simulink model "micro2018b"  (R2018b)
settings: Solver=ode1  StartTime=0.0  StopTime=t_sim  FixedStep=Ts  RelTol=1e-3
values from neighbouring files (symbols this model uses):
  Vo = 200    [param.m]
undefined symbols (not defined in the file or in its folder): C, f_i, fo, L, L1, L2, phi, R, Tm, Ts, Vac_pk
libraries: powerlib x16, powerlib_meascontrol x2, simulink x1, hdlsllib x1
(part 1 of 2)
settings Model: Creator=gomez  LastModifiedBy=gomez
settings DataIOCC: ReturnWorkspaceOutputs=on
settings DebuggingCC: UnconnectedInputMsg=none  UnconnectedOutputMsg=none  UnconnectedLineMsg=none  SFMachineParentedDataDiag=error

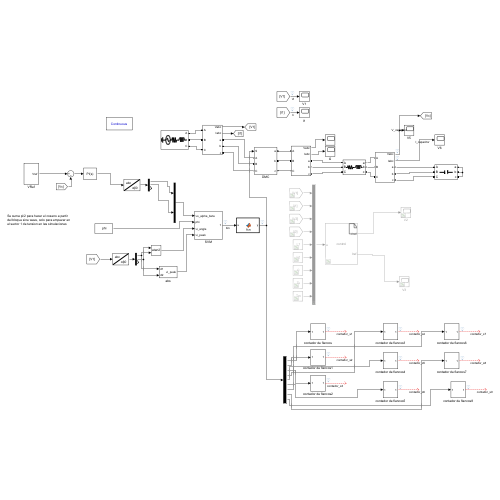
[thumbnail: Simulink's stored preview of the top-level diagram]
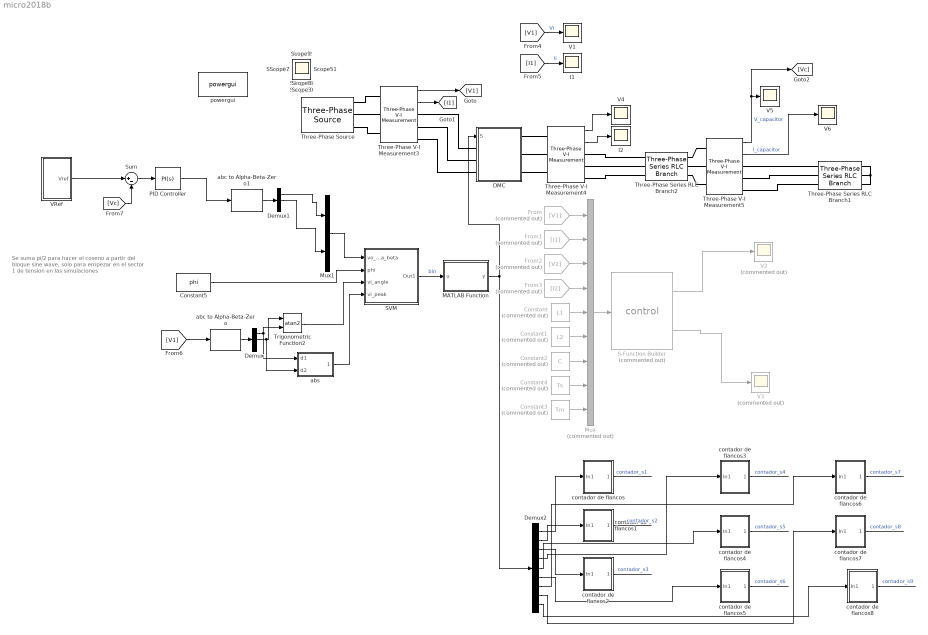
== system micro2018b ==
  note: Se suma pi/2 para hacer el coseno a partir del bloque sine wave, solo para empezar en el sector 1 de tension en las simulaciones
  Constant : Constant  Commented=on  Value=L1
  Constant1 : Constant  Commented=on  Value=L2
  Constant2 : Constant  Commented=on  Value=C
  Constant3 : Constant  Commented=on  Value=Tm
  Constant4 : Constant  Commented=on  Value=Ts
  Constant5 : Constant  Value=phi
  DMC : Subsystem
  Demux : Demux  Outputs=3
  Demux1 : Demux  Outputs=3
  Demux2 : Demux  Outputs=9
  From : From  Commented=on  GotoTag=V1
  From1 : From  Commented=on  GotoTag=I1
  From2 : From  Commented=on  GotoTag=V2
  From3 : From  Commented=on  GotoTag=I2
  I1 : Scope
  I2 : Scope
  MATLAB Function : MATLAB Function  TreatAsAtomicUnit=on
  Mux : Mux  Commented=on  Inputs=9
  Mux1 : Mux  Inputs=2
  PID Controller : simulink/Continuous/PID Controller  Controller=PI  Form=Parallel  TimeDomain=Continuous-time  SampleTime=-1  IntegratorMethod=Forward Euler  ControllerParametersSource=internal  P=1  I=1  D=0  N=100  UseFilter=on  TunerSelectOption=Transfer Function Based (PID Tuner App)  InitialConditionSource=internal  InitialConditionForIntegrator=0  InitialConditionForFilter=0  DifferentiatorICPrevScaledInput=0  ExternalReset=none  TrackingMode=off  Kt=1  LimitOutput=off  UpperSaturationLimit=inf  LowerSaturationLimit=-inf  LinearizeAsGain=on  AntiWindupMode=none  Kb=1  POutMin=[]  POutMax=[]  IOutMin=[]  IOutMax=[]  DOutMin=[]  DOutMax=[]  NOutMin=[]  NOutMax=[]  SumOutMin=[]  SumOutMax=[]  SaturationOutMin=[]  SaturationOutMax=[]  PParamMin=[]  PParamMax=[]  IParamMin=[]  IParamMax=[]  DParamMin=[]  DParamMax=[]  NParamMin=[]  NParamMax=[]  KbParamMin=[]  KbParamMax=[]  KtParamMin=[]  KtParamMax=[]  KbOutMin=[]  KbOutMax=[]  KtOutMin=[]  KtOutMax=[]  IntegratorOutMin=[]  IntegratorOutMax=[]  FilterOutMin=[]  FilterOutMax=[]  SumI1OutMin=[]  SumI1OutMax=[]  SumI2OutMin=[]  SumI2OutMax=[]  SumI3OutMin=[]  SumI3OutMax=[]  SumI4OutMin=[]  SumI4OutMax=[]  SumDOutMin=[]  SumDOutMax=[]  DifferentiatorOutMin=[]  DifferentiatorOutMax=[]  FilterDiffOutCoefMin=[]  FilterDiffOutCoefMax=[]  ReciprocalOutMin=[]  ReciprocalOutMax=[]  SumDenOutMin=[]  SumDenOutMax=[]  SumNumOutMin=[]  SumNumOutMax=[]  DivideOutMin=[]  DivideOutMax=[]  IntegratorContinuousStateAttributes=''  IntegratorStateMustResolveToSignalObject=off  IntegratorRTWStateStorageClass=Auto  FilterContinuousStateAttributes=''  FilterStateMustResolveToSignalObject=off  FilterRTWStateStorageClass=Auto  ParallelPVariant=InternalParameters  IdealPVariant=Disabled  IVariant=InternalParameters  DVariant=Disabled  IntegratorVariant=Continuous  SatVariant=Disabled  AWVariant=Passthrough  PCopyVariant=Disabled  TRVariant=Disabled  FdbkBlocksVariant=Forward  IdealPFdbkVariant=Disabled  SatFdbkVariant=Disabled  DerivativeFilterVariant=Disabled  NVariant=Disabled  NCopyVariant=Disabled_SignalSpec  FilterICVariant=Disabled  IntegratorICVariant=InternalICs  ExternalResetVariant=Disabled  TRSumVariant=Passthrough  SumFdbkVariant=Disabled  SumVariant=Sum_PI
  S-Function Builder : S-Function  Commented=on  FunctionName=control  SFunctionModules=control_wrapper  SFunctionDeploymentMode=off  EnableBusSupport=off  mask(S-Function Builder){}
      mask help: Simulink:masks:SFunctionBuilder_MD
      mask init:
      | val = [[.9  0.75 0.75 1 1 .9 .9 1]',[1 1 0.75 0.75 .9 .9 1 .9]'];try , sys = get_param(gcb,'SfunBuilderFcnName');if isempty(sys), sys = get_param(gcb,'FunctionName'); end,catch, sys = get_param(gcb,'FunctionName'); end
      settings: CopyFcn=set_param(gcbh,'LinkStatus','none')  OpenFcn=sfunctionwizard(gcbh)
      mask Display:
      | plot(val(:,1),val(:,2))
      | disp(sys)
      | port_label('input',1,'u')
      | port_label('output',1,'Vref')
      | port_label('output',2,'Iref')
  SVM : Subsystem
  Sum : Sum  Inputs=|+-
  Three-Phase Series RLC Branch1 : powerlib/Elements/Three-Phase Series RLC Branch  LConnTagsString=A|B|C  RConnTagsString=A|B|C  BranchType=C  Resistance=R  Inductance=L  Capacitance=C  Measurements=None
  Three-Phase Series RLC Branch2 : powerlib/Elements/Three-Phase Series RLC Branch  LConnTagsString=A|B|C  RConnTagsString=A|B|C  BranchType=RL  Resistance=R  Inductance=L  Capacitance=C  Measurements=None
  Three-Phase V-I Measurement3 : powerlib/Measurements/Three-Phase V-I Measurement  VoltageMeasurement=phase-to-ground  SetLabelV=off  LabelV=Vabc  Vpu=off  VpuLL=off  CurrentMeasurement=yes  SetLabelI=off  LabelI=Iabc  Ipu=off  Pbase=100e6  Vbase=500e3  OutputType=Complex  PhasorSimulation=off  PSBequivalent=0
  Three-Phase V-I Measurement4 : powerlib/Measurements/Three-Phase V-I Measurement  VoltageMeasurement=phase-to-ground  SetLabelV=off  LabelV=Vabc  Vpu=off  VpuLL=off  CurrentMeasurement=yes  SetLabelI=off  LabelI=Iabc  Ipu=off  Pbase=100e6  Vbase=500e3  OutputType=Complex  PhasorSimulation=off  PSBequivalent=0
  Three-Phase V-I Measurement5 : powerlib/Measurements/Three-Phase V-I Measurement  VoltageMeasurement=phase-to-ground  SetLabelV=off  LabelV=Vabc  Vpu=off  VpuLL=off  CurrentMeasurement=yes  SetLabelI=off  LabelI=Iabc  Ipu=off  Pbase=100e6  Vbase=500e3  OutputType=Complex  PhasorSimulation=off  PSBequivalent=0
  Three-Phase Source : powerlib/Electrical Sources/Three-Phase Source  InternalConnection=Yg  VoltagePhases=off  Voltage=Vac_pk  PhaseAngle=0  Voltage_phases=[25e3 25e3 25e3]/sqrt(3)  PhaseAngles_phases=[0 -120 +120]  Frequency=f_i  NonIdealSource=on  SpecifyImpedance=off  Resistance=0.1  Inductance=1e-3  ShortCircuitLevel=100e6  BaseVoltage=25e3  XRratio=7  BusType=swing  Pref=10e3  Qref=0  Prefabc=[10e3, 10e3, 10e3]  Qrefabc=[0, 0, 0]  Qmin=-inf  Qmax=inf
  Trigonometric Function2 : Trigonometry  Operator=atan2
  V{1,4..6} (4 alike) : Scope
  V2 : Scope  Commented=on
  V3 : Scope  Commented=on
  VRef : Subsystem
  abc to Alpha-Beta-Zero : powerlib_meascontrol/Transformations/abc to Alpha-Beta-Zero
  abc to Alpha-Beta-Zero1 : powerlib_meascontrol/Transformations/abc to Alpha-Beta-Zero
  abs : Subsystem
  contador de flancos : Subsystem
  contador de flancos1 : Subsystem
  contador de flancos2 : Subsystem
  contador de flancos3 : Subsystem
  contador de flancos4 : Subsystem
  contador de flancos5 : Subsystem
  contador de flancos6 : Subsystem
  contador de flancos7 : Subsystem
  contador de flancos8 : Subsystem
  powergui : powerlib/powergui  Priority=1  SimulationMode=Continuous  SampleTime=50e-6  frequency=60  Iterations=50  frequencyindice=50  Pbase=100e6  ErrMax=1e-4  UnitsV=kV  UnitsW=MW  buscounter=0  FunctionMessages=off  echomessages=off  EnableUseOfTLC=off  CurrentSourceSwitches=off  DisableSnubberDevices=off  DisableRonSwitches=off  DisableVfSwitches=off  DisplayEquations=off  AutomaticDiscreteSolvers=off  SolverType=Tustin/Backward Euler (TBE)  Interpol=off  ExternalGateDelay=off  methode=off  Ts=100  x0status=blocks  SPID=on  SwTol=0  HookPort=off  NonlinearTolerance=1e-4  nMaxIteration=100  ContinueOnMaxIteration=off  RestoreLinks=warning  ResistiveCurrentMeasurement=off  Frange=[0:2:500]  Ylog=off  Xlog=on  ShowGrid=off  save=off  variable=ZData  structure=0  ZoomFFT=off  StartTime=0.0  cycles=1  DisplayStyle=1  fundamental=60  FreqAxis=off  MaxFrequency=1000  frequencyindicesteady=1  RmsSteady=1  display=off
  Scope{,1..3,5,7..13} (12 alike) : Scope
  wires:
  Mux/1 -> S-Function Builder/1
  From/1 -> Mux/1
  From1/1 -> Mux/2
  From2/1 -> Mux/3
  From3/1 -> Mux/4
  Constant/1 -> Mux/5
  Constant1/1 -> Mux/6
  Constant2/1 -> Mux/7
  Constant4/1 -> Mux/8
  Constant3/1 -> Mux/9
  [V1] -> V1/1  "Vi"
  [I1] -> I1/1  "Ii"
  S-Function Builder/1 -> V2/1
  S-Function Builder/2 -> V3/1
  Constant5/1 -> SVM/2(phi)
  Demux1/1 -> Mux1/1
  Demux1/2 -> Mux1/2
  Mux1/1 -> SVM/1(vo_alpha_beta)
  SVM/1(Out1) -> MATLAB Function/1(u)  "bin"
  [V1] -> abc to Alpha-Beta-Zero/1
  abc to Alpha-Beta-Zero/1 -> Demux/1
  Demux/2 -> abs/2(d2), Trigonometric Function2/1
  Demux/1 -> Trigonometric Function2/2, abs/1(d1)
  Trigonometric Function2/1 -> SVM/3(vi_angle)
  abs/1(vi_peak) -> SVM/4(vi_peak)
  Three-Phase V-I Measurement4/1 -> V4/1
  Three-Phase V-I Measurement4/2 -> I2/1
  MATLAB Function/1(y) -> Demux2/1, DMC/1(S)
  Three-Phase V-I Measurement3/1 -> [V1]
  Three-Phase V-I Measurement3/2 -> [I1]
  Three-Phase V-I Measurement5/1 -> [Vc], V5/1  "V_capacitor"
  Three-Phase V-I Measurement5/2 -> V6/1  "I_capacitor"
  abc to Alpha-Beta-Zero1/1 -> Demux1/1
  Demux2/1 -> contador de flancos/1(In1)
  contador de flancos/1(Out1) -> ?  "contador_s1"
  contador de flancos1/1(Out1) -> ?  "contador_s2"
  Demux2/2 -> contador de flancos1/1(In1)
  contador de flancos2/1(Out1) -> ?  "contador_s3"
  Demux2/3 -> contador de flancos2/1(In1)
  contador de flancos3/1(Out1) -> ?  "contador_s4"
  Demux2/4 -> contador de flancos3/1(In1)
  contador de flancos4/1(Out1) -> ?  "contador_s5"
  Demux2/5 -> contador de flancos4/1(In1)
  contador de flancos5/1(Out1) -> ?  "contador_s6"
  Demux2/6 -> contador de flancos5/1(In1)
  contador de flancos6/1(Out1) -> ?  "contador_s7"
  Demux2/7 -> contador de flancos6/1(In1)
  contador de flancos7/1(Out1) -> ?  "contador_s8"
  Demux2/8 -> contador de flancos7/1(In1)
  contador de flancos8/1(Out1) -> ?  "contador_s9"
  Demux2/9 -> contador de flancos8/1(In1)
  VRef/1(Vref) -> Sum/1
  [Vc] -> Sum/2
  Sum/1 -> PID Controller/1
  PID Controller/1 -> abc to Alpha-Beta-Zero1/1
  connections:
  Three-Phase V-I Measurement4/RConn1 -- Three-Phase Series RLC Branch2/LConn1
  Three-Phase Source/RConn1 -- Three-Phase V-I Measurement3/LConn1
  Three-Phase Source/RConn3 -- Three-Phase V-I Measurement3/LConn3
  Three-Phase V-I Measurement4/LConn1 -- DMC/RConn1
  Three-Phase V-I Measurement4/LConn2 -- DMC/RConn2
  Three-Phase V-I Measurement4/LConn3 -- DMC/RConn3
  Three-Phase Series RLC Branch2/LConn2 -- Three-Phase V-I Measurement4/RConn2
  Three-Phase Series RLC Branch2/LConn3 -- Three-Phase V-I Measurement4/RConn3
  Three-Phase Source/RConn2 -- Three-Phase V-I Measurement3/LConn2
  Three-Phase V-I Measurement3/RConn2 -- DMC/LConn2
  Three-Phase V-I Measurement3/RConn1 -- DMC/LConn1
  Three-Phase V-I Measurement3/RConn3 -- DMC/LConn3
  Three-Phase V-I Measurement5/RConn1 -- Three-Phase Series RLC Branch1/LConn1
  Three-Phase V-I Measurement5/RConn2 -- Three-Phase Series RLC Branch1/LConn2
  Three-Phase V-I Measurement5/RConn3 -- Three-Phase Series RLC Branch1/LConn3
  Three-Phase Series RLC Branch1/RConn1 -- Three-Phase Series RLC Branch1/RConn2 -- Three-Phase Series RLC Branch1/RConn3
  Three-Phase Series RLC Branch2/RConn2 -- Three-Phase V-I Measurement5/LConn2
  Three-Phase V-I Measurement5/LConn1 -- Three-Phase Series RLC Branch2/RConn1
  Three-Phase V-I Measurement5/LConn3 -- Three-Phase Series RLC Branch2/RConn3

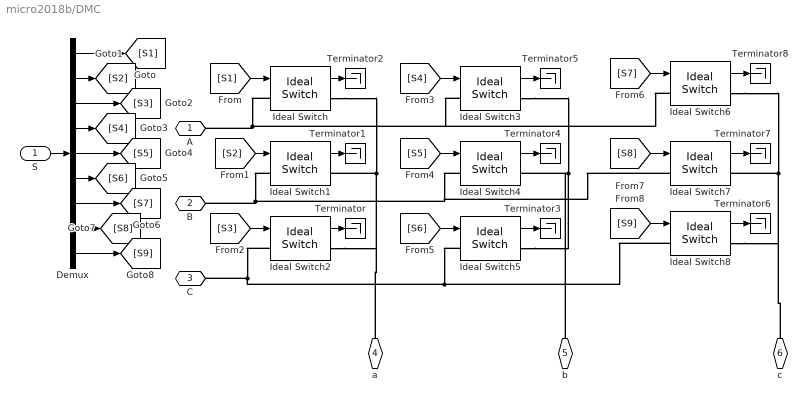
== system micro2018b/DMC ==
  S : Inport
  Demux : Demux  Outputs=9
  Ideal Switch{,1..8} (9 alike) : powerlib/Power Electronics/Ideal Switch  Ron=0.001  Lon=0  IC=0  Rs=1e5  Cs=inf  Measurements=on
  Terminator{,1..8} (9 alike) : Terminator
  A : PMIOPort  Side=Left
  B : PMIOPort  Port=2  Side=Left
  C : PMIOPort  Port=3  Side=Left
  a : PMIOPort  Port=4  Side=Right
  b : PMIOPort  Port=5  Side=Right
  c : PMIOPort  Port=6  Side=Right
  wires:
  [S8] -> Ideal Switch7/1
  Ideal Switch4/1 -> Terminator4/1
  Ideal Switch/1 -> Terminator2/1
  Ideal Switch7/1 -> Terminator7/1
  Ideal Switch8/1 -> Terminator6/1
  Ideal Switch3/1 -> Terminator5/1
  Ideal Switch6/1 -> Terminator8/1
  Ideal Switch2/1 -> Terminator/1
  Ideal Switch1/1 -> Terminator1/1
  [S4] -> Ideal Switch3/1
  [S3] -> Ideal Switch2/1
  Ideal Switch5/1 -> Terminator3/1
  [S2] -> Ideal Switch1/1
  [S9] -> Ideal Switch8/1
  [S6] -> Ideal Switch5/1
  [S5] -> Ideal Switch4/1
  [S1] -> Ideal Switch/1
  Demux/1 -> [S1]
  Demux/2 -> [S2]
  Demux/3 -> [S3]
  Demux/4 -> [S4]
  Demux/5 -> [S5]
  Demux/6 -> [S6]
  Demux/7 -> [S7]
  Demux/8 -> [S8]
  Demux/9 -> [S9]
  [S7] -> Ideal Switch6/1
  S/1 -> Demux/1
  connections:
  Ideal Switch1/LConn1 -- Ideal Switch4/LConn1 -- Ideal Switch7/LConn1 -- B/RConn1
  Ideal Switch/RConn1 -- a/RConn1 -- Ideal Switch2/RConn1 -- Ideal Switch1/RConn1
  Ideal Switch6/RConn1 -- Ideal Switch7/RConn1 -- c/RConn1 -- Ideal Switch8/RConn1
  Ideal Switch8/LConn1 -- Ideal Switch2/LConn1 -- C/RConn1 -- Ideal Switch5/LConn1
  Ideal Switch/LConn1 -- Ideal Switch6/LConn1 -- Ideal Switch3/LConn1 -- A/RConn1
  Ideal Switch3/RConn1 -- b/RConn1 -- Ideal Switch5/RConn1 -- Ideal Switch4/RConn1

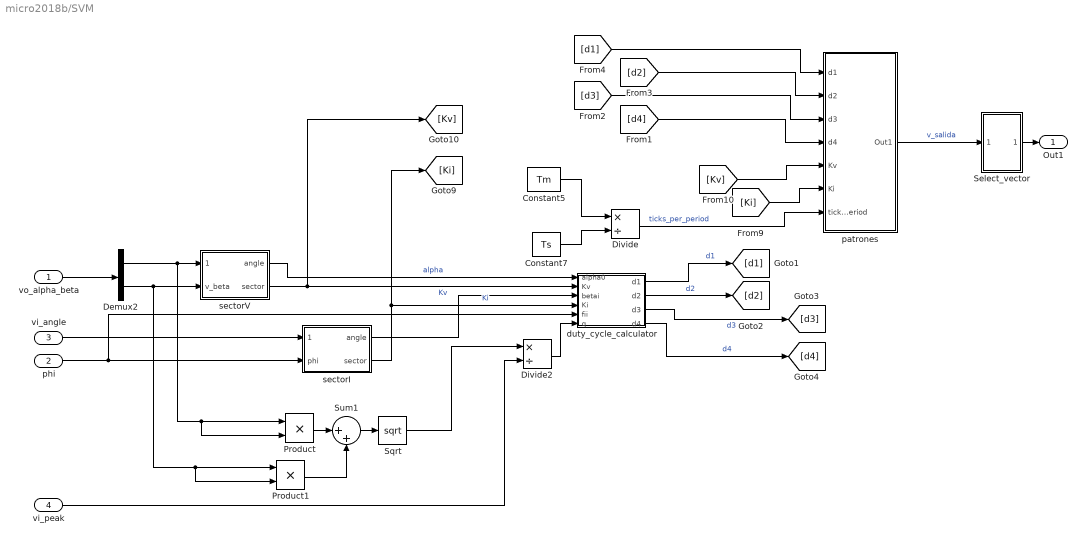
== system micro2018b/SVM ==
  vo_alpha_beta : Inport
  phi : Inport  Port=2
  vi_angle : Inport  Port=3
  vi_peak : Inport  Port=4
  Constant5 : Constant  Value=Tm
  Constant7 : Constant  Value=Ts
  Demux2 : Demux  Outputs=2
  Divide : Product  Inputs=*/
  Divide2 : Product  Inputs=*/
  Product : Product
  Product1 : Product
  Select_vector : Subsystem
  Sqrt : Sqrt  SaturateOnIntegerOverflow=on
  Sum1 : Sum  Inputs=|++
  duty_cycle_calculator : MATLAB Function  TreatAsAtomicUnit=on
  patrones : Subsystem
  sectorI : MATLAB Function  TreatAsAtomicUnit=on
  sectorV : MATLAB Function  TreatAsAtomicUnit=on
  Out1 : Outport
  wires:
  Sqrt/1 -> Divide2/1
  duty_cycle_calculator/4(d4) -> [d4]  "d4"
  sectorV/1(angle) -> duty_cycle_calculator/1(alpha0)  "alpha"
  duty_cycle_calculator/3(d3) -> [d3]  "d3"
  Demux2/2 -> Product1/2, Product1/1, sectorV/2(v_beta)
  vo_alpha_beta/1 -> Demux2/1
  Demux2/1 -> Product/2, Product/1, sectorV/1(v_alpha)
  sectorV/2(sector) -> [Kv], duty_cycle_calculator/2(Kv)  "Kv"
  duty_cycle_calculator/2(d2) -> [d2]  "d2"
  duty_cycle_calculator/1(d1) -> [d1]  "d1"
  Divide2/1 -> duty_cycle_calculator/6(q)
  Product1/1 -> Sum1/2
  phi/1 -> duty_cycle_calculator/5(fii), sectorI/2(phi)
  sectorI/2(sector) -> [Ki], duty_cycle_calculator/4(Ki)  "Ki"
  sectorI/1(angle) -> duty_cycle_calculator/3(betai)
  Sum1/1 -> Sqrt/1
  Product/1 -> Sum1/1
  vi_angle/1 -> sectorI/1(Vi_angle)
  vi_peak/1 -> Divide2/2
  Select_vector/1(Out1) -> Out1/1
  [d1] -> patrones/1(d1)
  [d2] -> patrones/2(d2)
  [d3] -> patrones/3(d3)
  [d4] -> patrones/4(d4)
  [Ki] -> patrones/6(Ki)
  [Kv] -> patrones/5(Kv)
  patrones/1(Out1) -> Select_vector/1(In1)  "v_salida"
  Constant5/1 -> Divide/1
  Constant7/1 -> Divide/2
  Divide/1 -> patrones/7(ticks_per_period)  "ticks_per_period"

== system micro2018b/VRef ==
  Mux : Mux  Inputs=3
  VA : Sin  Amplitude=Vo  Frequency=2*pi*fo  SampleTime=0
  VB : Sin  Amplitude=Vo  Frequency=2*pi*fo  Phase=-2*pi/3  SampleTime=0
  VC : Sin  Amplitude=Vo  Frequency=2*pi*fo  Phase=-4*pi/3  SampleTime=0
  Vref : Outport  VectorParamsAs1DForOutWhenUnconnected=off
  wires:
  VA/1 -> Mux/1
  VB/1 -> Mux/2
  VC/1 -> Mux/3
  Mux/1 -> Vref/1

== system micro2018b/abs ==
  d1 : Inport
  d2 : Inport  Port=2
  Add : Sum
  Product1 : Product
  Product2 : Product
  Sqrt1 : Sqrt  SaturateOnIntegerOverflow=on
  vi_peak : Outport
  wires:
  d1/1 -> Product2/2, Product2/1
  Sqrt1/1 -> vi_peak/1
  d2/1 -> Product1/2, Product1/1
  Product1/1 -> Add/2
  Product2/1 -> Add/1
  Add/1 -> Sqrt1/1

== system micro2018b/contador de flancos ==
  In1 : Inport
  Add : Sum
  Data Type Conversion : DataTypeConversion
  Delay : Delay  DelayLength=1
  Delay1 : Delay  DelayLength=1
  Relational Operator : RelationalOperator  Operator=>  OutDataTypeStr=boolean  RndMeth=Simplest
  Out1 : Outport
  wires:
  In1/1 -> Delay/1, Relational Operator/1
  Relational Operator/1 -> Data Type Conversion/1
  Delay1/1 -> Add/2, Out1/1
  Add/1 -> Delay1/1
  Delay/1 -> Relational Operator/2
  Data Type Conversion/1 -> Add/1

== system micro2018b/contador de flancos1 ==
  In1 : Inport
  Add : Sum
  Data Type Conversion : DataTypeConversion
  Delay : Delay  DelayLength=1
  Delay1 : Delay  DelayLength=1
  Relational Operator : RelationalOperator  Operator=>  OutDataTypeStr=boolean  RndMeth=Simplest
  Out1 : Outport
  wires:
  In1/1 -> Delay/1, Relational Operator/1
  Relational Operator/1 -> Data Type Conversion/1
  Delay1/1 -> Out1/1, Add/2
  Add/1 -> Delay1/1
  Delay/1 -> Relational Operator/2
  Data Type Conversion/1 -> Add/1

== system micro2018b/contador de flancos2 ==
  In1 : Inport
  Add : Sum
  Data Type Conversion1 : DataTypeConversion
  Delay : Delay  DelayLength=1
  Delay1 : Delay  DelayLength=1
  Relational Operator : RelationalOperator  Operator=>  OutDataTypeStr=boolean  RndMeth=Simplest
  Out1 : Outport
  wires:
  In1/1 -> Delay/1, Relational Operator/1
  Relational Operator/1 -> Data Type Conversion1/1
  Delay1/1 -> Out1/1, Add/2
  Add/1 -> Delay1/1
  Delay/1 -> Relational Operator/2
  Data Type Conversion1/1 -> Add/1

== system micro2018b/contador de flancos3 ==
  In1 : Inport
  Add : Sum
  Data Type Conversion : DataTypeConversion
  Delay : Delay  DelayLength=1
  Delay1 : Delay  DelayLength=1
  Relational Operator : RelationalOperator  Operator=>  OutDataTypeStr=boolean  RndMeth=Simplest
  Out1 : Outport
  wires:
  In1/1 -> Delay/1, Relational Operator/1
  Relational Operator/1 -> Data Type Conversion/1
  Delay1/1 -> Out1/1, Add/2
  Add/1 -> Delay1/1
  Delay/1 -> Relational Operator/2
  Data Type Conversion/1 -> Add/1

== system micro2018b/contador de flancos4 ==
  In1 : Inport
  Add : Sum
  Data Type Conversion : DataTypeConversion
  Delay : Delay  DelayLength=1
  Delay1 : Delay  DelayLength=1
  Relational Operator : RelationalOperator  Operator=>  OutDataTypeStr=boolean  RndMeth=Simplest
  Out1 : Outport
  wires:
  In1/1 -> Delay/1, Relational Operator/1
  Relational Operator/1 -> Data Type Conversion/1
  Delay1/1 -> Out1/1, Add/2
  Add/1 -> Delay1/1
  Delay/1 -> Relational Operator/2
  Data Type Conversion/1 -> Add/1

== system micro2018b/contador de flancos5 ==
  In1 : Inport
  Add : Sum
  Data Type Conversion : DataTypeConversion
  Delay : Delay  DelayLength=1
  Delay1 : Delay  DelayLength=1
  Relational Operator : RelationalOperator  Operator=>  OutDataTypeStr=boolean  RndMeth=Simplest
  Out1 : Outport
  wires:
  In1/1 -> Delay/1, Relational Operator/1
  Relational Operator/1 -> Data Type Conversion/1
  Delay1/1 -> Out1/1, Add/2
  Add/1 -> Delay1/1
  Delay/1 -> Relational Operator/2
  Data Type Conversion/1 -> Add/1

== system micro2018b/contador de flancos6 ==
  In1 : Inport
  Add : Sum
  Data Type Conversion : DataTypeConversion
  Delay : Delay  DelayLength=1
  Delay1 : Delay  DelayLength=1
  Relational Operator : RelationalOperator  Operator=>  OutDataTypeStr=boolean  RndMeth=Simplest
  Out1 : Outport
  wires:
  In1/1 -> Delay/1, Relational Operator/1
  Relational Operator/1 -> Data Type Conversion/1
  Delay1/1 -> Out1/1, Add/2
  Add/1 -> Delay1/1
  Delay/1 -> Relational Operator/2
  Data Type Conversion/1 -> Add/1

== system micro2018b/contador de flancos7 ==
  In1 : Inport
  Add : Sum
  Data Type Conversion : DataTypeConversion
  Delay : Delay  DelayLength=1
  Delay1 : Delay  DelayLength=1
  Relational Operator : RelationalOperator  Operator=>  OutDataTypeStr=boolean  RndMeth=Simplest
  Out1 : Outport
  wires:
  In1/1 -> Delay/1, Relational Operator/1
  Relational Operator/1 -> Data Type Conversion/1
  Delay1/1 -> Out1/1, Add/2
  Add/1 -> Delay1/1
  Delay/1 -> Relational Operator/2
  Data Type Conversion/1 -> Add/1

== system micro2018b/contador de flancos8 ==
  In1 : Inport
  Add : Sum
  Data Type Conversion : DataTypeConversion
  Delay : Delay  DelayLength=1
  Delay1 : Delay  DelayLength=1
  Relational Operator : RelationalOperator  Operator=>  OutDataTypeStr=boolean  RndMeth=Simplest
  Out1 : Outport
  wires:
  In1/1 -> Delay/1, Relational Operator/1
  Relational Operator/1 -> Data Type Conversion/1
  Delay1/1 -> Out1/1, Add/2
  Add/1 -> Delay1/1
  Delay/1 -> Relational Operator/2
  Data Type Conversion/1 -> Add/1

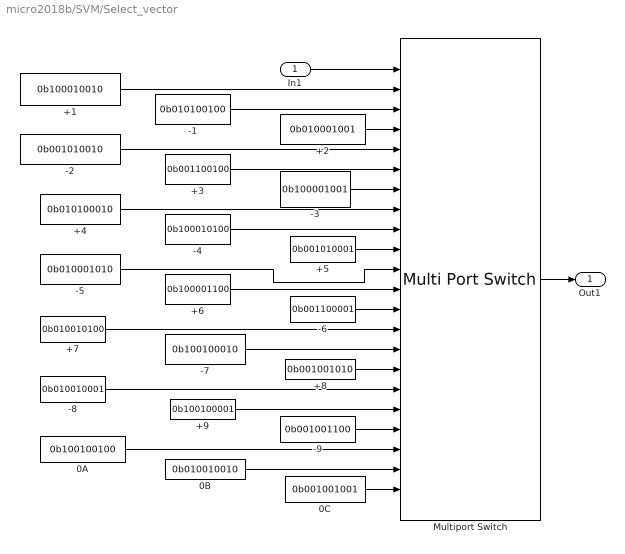
== system micro2018b/SVM/Select_vector ==
  In1 : Inport
  +1 : Constant  Value=0b100010010
  +2 : Constant  Value=0b010001001
  +3 : Constant  Value=0b001100100
  +4 : Constant  Value=0b010100010
  +5 : Constant  Value=0b001010001
  +6 : Constant  Value=0b100001100
  +7 : Constant  Value=0b010010100
  +8 : Constant  Value=0b001001010
  +9 : Constant  Value=0b100100001
  -1 : Constant  Value=0b010100100
  -2 : Constant  Value=0b001010010
  -3 : Constant  Value=0b100001001
  -4 : Constant  Value=0b100010100
  -5 : Constant  Value=0b010001010
  -6 : Constant  Value=0b001100001
  -7 : Constant  Value=0b100100010
  -8 : Constant  Value=0b010010001
  -9 : Constant  Value=0b001001100
  0A : Constant  Value=0b100100100
  0B : Constant  Value=0b010010010
  0C : Constant  Value=0b001001001
  Multiport Switch : MultiPortSwitch  DataPortOrder=Specify indices  Inputs=21  DataPortIndices={1,-1,2,-2,3,-3,4,-4,5,-5,6,-6,7,-7,8,-8,9,-9,19,20,21}  DiagnosticForDefault=Warning
  Out1 : Outport
  wires:
  +7/1 -> Multiport Switch/14
  -8/1 -> Multiport Switch/17
  +4/1 -> Multiport Switch/8
  In1/1 -> Multiport Switch/1
  +3/1 -> Multiport Switch/6
  +9/1 -> Multiport Switch/18
  +2/1 -> Multiport Switch/4
  -4/1 -> Multiport Switch/9
  -5/1 -> Multiport Switch/11
  -7/1 -> Multiport Switch/15
  -1/1 -> Multiport Switch/3
  -2/1 -> Multiport Switch/5
  -6/1 -> Multiport Switch/13
  +5/1 -> Multiport Switch/10
  -9/1 -> Multiport Switch/19
  +1/1 -> Multiport Switch/2
  +8/1 -> Multiport Switch/16
  +6/1 -> Multiport Switch/12
  -3/1 -> Multiport Switch/7
  Multiport Switch/1 -> Out1/1
  0C/1 -> Multiport Switch/22
  0B/1 -> Multiport Switch/21
  0A/1 -> Multiport Switch/20

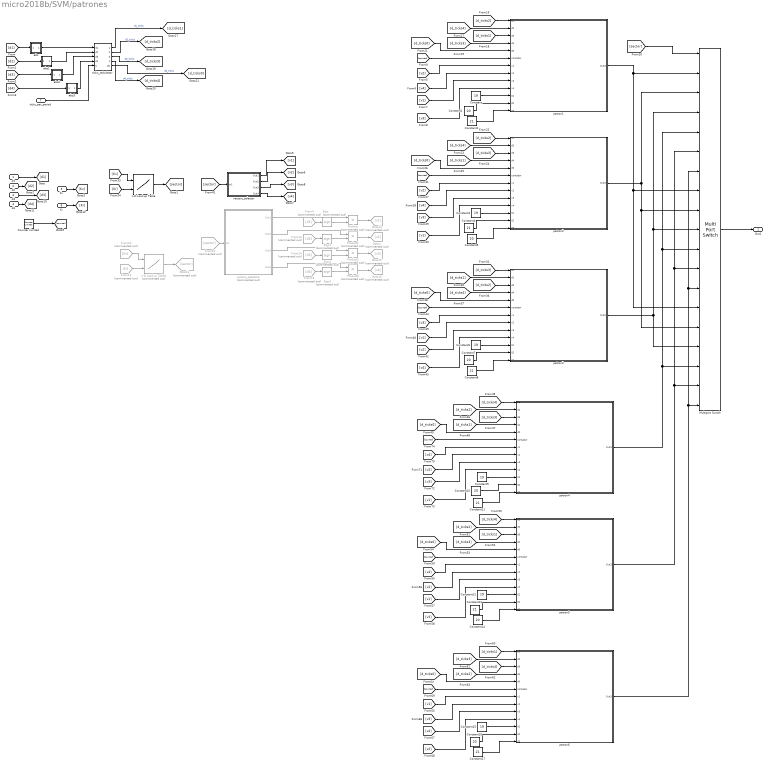
== system micro2018b/SVM/patrones ==
  d1 : Inport
  d2 : Inport  Port=2
  d3 : Inport  Port=3
  d4 : Inport  Port=4
  Kv : Inport  Port=5
  Ki : Inport  Port=6
  ticks_per_period : Inport  Port=7
  Constant{,3,6,9,12,15} (6 alike) : Constant  Value=19
  Constant{1,5,7,10,14,16} (6 alike) : Constant  Value=20
  Constant{2,4,8,11,13,17} (6 alike) : Constant  Value=21
  Counter Limited : hdlsllib/Sources/Counter Limited  uplimit=Tm/Ts  tsamp=-1
      settings: SourceProductBaseCode=SL
  From10 : From  Commented=on  GotoTag=Kv
  From11 : From  Commented=on  GotoTag=Ki
  From12 : From  Commented=on  GotoTag=sector
  From13 : From  Commented=on  GotoTag=d2
  From14 : From  Commented=on  GotoTag=d3
  From15 : From  Commented=on  GotoTag=d4
  From4 : From  Commented=on  GotoTag=d1
  Goto13 : Goto  Commented=on  GotoTag=sector
  Goto14 : Goto  Commented=on  GotoTag=v1
  Goto15 : Goto  Commented=on  GotoTag=v3
  Goto16 : Goto  Commented=on  GotoTag=v4
  Goto4 : Goto  Commented=on  GotoTag=v2
  Multiport Switch : MultiPortSwitch  Inputs=18
  Product{,1..3} (4 alike) : Product  Commented=on
  Sign{,1..3} (4 alike) : Signum  Commented=on
  abs : Subsystem
  abs1 : Subsystem
  abs2 : Subsystem
  abs3 : Subsystem
  n-D Lookup Table : Lookup_n-D  LookupTableObject=''  BreakpointsForDimension1=[1;2;3;4;5;6]  BreakpointsForDimension2=[1;2;3;4;5;6]  BreakpointsForDimension3=[5, 7]  BreakpointsForDimension1FirstPoint=10  BreakpointsForDimension2FirstPoint=10  BreakpointsForDimension1Spacing=12  BreakpointsForDimension2Spacing=12  IndexSearchMethod=Evenly spaced points  Table=[1 2 3 10 11 12;4 5 6 13 14 15;7 8 9 16 17 18;10 11 12 1 2 3;13 14 15 4 5 6;16 17 18 7 8 9]  InterpMethod=Flat  DiagnosticForOutOfRangeInput=Warning  InternalRulePriority=Speed  RndMeth=Simplest  InputSameDT=on
  n-D Lookup Table1 : Lookup_n-D  Commented=on  LookupTableObject=''  BreakpointsForDimension1=[1;2;3;4;5;6]  BreakpointsForDimension2=[1;2;3;4;5;6]  BreakpointsForDimension3=[5, 7]  BreakpointsForDimension1FirstPoint=10  BreakpointsForDimension2FirstPoint=10  BreakpointsForDimension1Spacing=12  BreakpointsForDimension2Spacing=12  IndexSearchMethod=Evenly spaced points  Table=[1 2 3 1 2 3;4 5 6 4 5 6;7 8 9 7 8 9;1 2 3 1 2 3;4 5 6 4 5 6;7 8 9 7 8 9]  InterpMethod=Flat  DiagnosticForOutOfRangeInput=Warning  InternalRulePriority=Speed  RndMeth=Simplest  InputSameDT=on
  patron1 : Subsystem
  patron2 : Subsystem
  patron3 : Subsystem
  patron4 : Subsystem
  patron5 : Subsystem
  patron6 : Subsystem
  ticks_calculator : Subsystem
  vectors_selector : Subsystem
  vectors_selector1 : Subsystem  Commented=on
  Out1 : Outport
  wires:
  Counter Limited/1 -> [counter]
  [d2] -> abs1/1(In1)
  [d3] -> abs2/1(In1)
  [d4] -> abs3/1(In1)
  ticks_calculator/5(d0) -> [d_ticks0]  "d0_ticks"
  [counter] -> patron1/6(contador)
  Kv/1 -> [Kv]
  d2/1 -> [d2]
  d1/1 -> [d1]
  d3/1 -> [d3]
  d4/1 -> [d4]
  Ki/1 -> [Ki]
  n-D Lookup Table/1 -> [sector]
  [Kv] -> n-D Lookup Table/1
  [Ki] -> n-D Lookup Table/2
  [sector] -> vectors_selector/1(In1)
  vectors_selector/1(Out1) -> [v1]
  vectors_selector/2(Out2) -> [v2]
  vectors_selector/3(Out3) -> [v3]
  vectors_selector/4(Out4) -> [v4]
  patron1/1(Out3) -> Multiport Switch/2, Multiport Switch/14, Multiport Switch/8
  [v2] -> patron1/7(v1)
  [v4] -> patron1/8(v2)
  [v3] -> patron1/10(v4)
  [v1] -> patron1/9(v3)
  Constant/1 -> patron1/11(01)
  Constant1/1 -> patron1/12(02)
  Constant2/1 -> patron1/13(03)
  From11/1 -> n-D Lookup Table1/2
  From10/1 -> n-D Lookup Table1/1
  n-D Lookup Table1/1 -> Goto13/1
  From12/1 -> vectors_selector1/1(In1)
  ticks_per_period/1 -> ticks_calculator/5(ticks_per_period)
  From4/1 -> Sign/1
  vectors_selector1/1(Out1) -> Product/1
  Sign/1 -> Product/2
  Product/1 -> Goto14/1
  From13/1 -> Sign1/1
  Sign1/1 -> Product1/2
  Product1/1 -> Goto4/1
  vectors_selector1/2(Out2) -> Product1/1
  From14/1 -> Sign2/1
  Sign2/1 -> Product2/2
  Product2/1 -> Goto15/1
  vectors_selector1/3(Out3) -> Product2/1
  From15/1 -> Sign3/1
  Sign3/1 -> Product3/2
  Product3/1 -> Goto16/1
  vectors_selector1/4(Out4) -> Product3/1
  [d1] -> abs/1(In1)
  abs/1(Out1) -> ticks_calculator/1(d1)
  abs1/1(Out1) -> ticks_calculator/2(d2)
  abs2/1(Out1) -> ticks_calculator/3(d3)
  abs3/1(Out1) -> ticks_calculator/4(d4)
  ticks_calculator/1(Out1) -> [d_ticks1]  "d1_ticks"
  ticks_calculator/2(Out2) -> [d_ticks2]  "d2_ticks"
  ticks_calculator/3(Out3) -> [d_ticks3]  "d3_ticks"
  ticks_calculator/4(Out4) -> [d_ticks4]  "d4_ticks"
  [d_ticks2] -> patron1/1(d1)
  [d_ticks4] -> patron1/2(d2)
  [d_ticks1] -> patron1/3(d3)
  [d_ticks3] -> patron1/4(d4)
  [sector] -> Multiport Switch/1
  Multiport Switch/1 -> Out1/1
  [d_ticks0] -> patron1/5(d0)
  [d_ticks3] -> patron2/3(d3)
  Constant3/1 -> patron2/11(01)
  Constant5/1 -> patron2/13(03)
  Constant4/1 -> patron2/12(02)
  [d_ticks2] -> patron2/1(d1)
  [counter] -> patron2/6(contador)
  [d_ticks4] -> patron2/2(d2)
  [v1] -> patron2/10(v4)
  [v4] -> patron2/8(v2)
  [d_ticks1] -> patron2/4(d4)
  [d_ticks0] -> patron2/5(d0)
  [v2] -> patron2/7(v1)
  [v3] -> patron2/9(v3)
  patron2/1(Out3) -> Multiport Switch/9, Multiport Switch/15, Multiport Switch/3
  [v2] -> patron3/9(v3)
  [v1] -> patron3/8(v2)
  [v3] -> patron3/7(v1)
  [d_ticks0] -> patron3/5(d0)
  [v4] -> patron3/10(v4)
  Constant7/1 -> patron3/12(02)
  Constant8/1 -> patron3/13(03)
  [d_ticks4] -> patron3/4(d4)
  [d_ticks1] -> patron3/2(d2)
  [d_ticks3] -> patron3/1(d1)
  Constant6/1 -> patron3/11(01)
  [d_ticks2] -> patron3/3(d3)
  [counter] -> patron3/6(contador)
  patron3/1(Out3) -> Multiport Switch/16, Multiport Switch/10, Multiport Switch/4
  [v1] -> patron5/9(v3)
  [v2] -> patron5/8(v2)
  Constant11/1 -> patron4/13(03)
  [v4] -> patron5/7(v1)
  [d_ticks3] -> patron5/4(d4)
  Constant13/1 -> patron5/12(02)
  Constant14/1 -> patron5/13(03)
  [d_ticks2] -> patron5/2(d2)
  [d_ticks4] -> patron5/1(d1)
  Constant10/1 -> patron4/12(02)
  Constant12/1 -> patron5/11(01)
  [d_ticks1] -> patron4/4(d4)
  [counter] -> patron5/6(contador)
  [d_ticks0] -> patron4/5(d0)
  [v3] -> patron4/9(v3)
  [d_ticks4] -> patron4/1(d1)
  [counter] -> patron4/6(contador)
  [v1] -> patron4/10(v4)
  [d_ticks4] -> patron6/3(d3)
  [counter] -> patron6/6(contador)
  [d_ticks2] -> patron6/4(d4)
  [d_ticks0] -> patron5/5(d0)
  Constant17/1 -> patron6/13(03)
  [d_ticks1] -> patron5/3(d3)
  Constant16/1 -> patron6/12(02)
  [v2] -> patron6/10(v4)
  Constant9/1 -> patron4/11(01)
  [d_ticks0] -> patron6/5(d0)
  [v1] -> patron6/7(v1)
  [v3] -> patron5/10(v4)
  [v3] -> patron6/8(v2)
  [v4] -> patron6/9(v3)
  Constant15/1 -> patron6/11(01)
  [d_ticks3] -> patron6/2(d2)
  [d_ticks3] -> patron4/3(d3)
  [d_ticks2] -> patron4/2(d2)
  [d_ticks1] -> patron6/1(d1)
  [v2] -> patron4/8(v2)
  [v4] -> patron4/7(v1)
  patron4/1(Out3) -> Multiport Switch/17, Multiport Switch/11, Multiport Switch/5
  patron5/1(Out3) -> Multiport Switch/18, Multiport Switch/12, Multiport Switch/6
  patron6/1(Out3) -> Multiport Switch/13, Multiport Switch/7, Multiport Switch/19

== system micro2018b/SVM/patrones/abs ==
  In1 : Inport
  Product4 : Product
  Sqrt : Sqrt  SaturateOnIntegerOverflow=on
  Out1 : Outport
  wires:
  In1/1 -> Product4/1, Product4/2
  Product4/1 -> Sqrt/1
  Sqrt/1 -> Out1/1

== system micro2018b/SVM/patrones/abs1 ==
  In1 : Inport
  Product4 : Product
  Sqrt : Sqrt  SaturateOnIntegerOverflow=on
  Out1 : Outport
  wires:
  In1/1 -> Product4/1, Product4/2
  Product4/1 -> Sqrt/1
  Sqrt/1 -> Out1/1

== system micro2018b/SVM/patrones/abs2 ==
  In1 : Inport
  Product4 : Product
  Sqrt : Sqrt  SaturateOnIntegerOverflow=on
  Out1 : Outport
  wires:
  In1/1 -> Product4/1, Product4/2
  Product4/1 -> Sqrt/1
  Sqrt/1 -> Out1/1

== system micro2018b/SVM/patrones/abs3 ==
  In1 : Inport
  Product4 : Product
  Sqrt : Sqrt  SaturateOnIntegerOverflow=on
  Out1 : Outport
  wires:
  In1/1 -> Product4/1, Product4/2
  Product4/1 -> Sqrt/1
  Sqrt/1 -> Out1/1

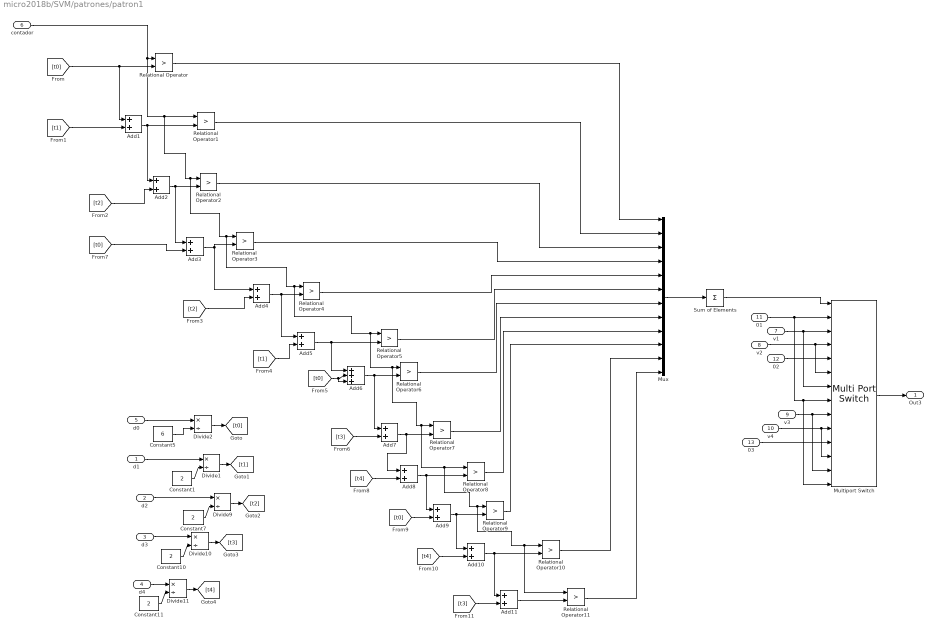
== system micro2018b/SVM/patrones/patron1 ==
  d1 : Inport
  d2 : Inport  Port=2
  d3 : Inport  Port=3
  d4 : Inport  Port=4
  d0 : Inport  Port=5
  contador : Inport  Port=6
  v1 : Inport  Port=7
  v2 : Inport  Port=8
  v3 : Inport  Port=9
  v4 : Inport  Port=10
  01 : Inport  Port=11
  02 : Inport  Port=12
  03 : Inport  Port=13
  Add{1..5,7..11} (10 alike) : Sum
  Add6 : Sum  Inputs=+++
  Constant{1,7,10..11} (4 alike) : Constant  Value=2
  Constant5 : Constant  Value=6
  Divide{1..2,9..11} (5 alike) : Product  Inputs=*/
  Multiport Switch : MultiPortSwitch  DataPortOrder=Zero-based contiguous  Inputs=13  zeroidx=on
  Mux : Mux  Inputs=12
  Relational Operator{,1..11} (12 alike) : RelationalOperator  Operator=>  OutDataTypeStr=boolean  RndMeth=Simplest
  Sum of Elements : Sum  Inputs=+
  Out3 : Outport
  wires:
  contador/1 -> Relational Operator11/1, Relational Operator10/1, Relational Operator9/1, Relational Operator8/1, Relational Operator7/1, Relational Operator6/1, Relational Operator5/1, Relational Operator4/1, Relational Operator3/1, Relational Operator2/1, Relational Operator1/1, Relational Operator/1
  Add10/1 -> Add11/1, Relational Operator10/2
  Add9/1 -> Add10/1, Relational Operator9/2
  [t2] -> Add4/2
  Relational Operator8/1 -> Mux/9
  [t0] -> Add1/1, Relational Operator/2
  Relational Operator/1 -> Mux/1
  Relational Operator1/1 -> Mux/2
  Relational Operator5/1 -> Mux/6
  Add2/1 -> Add3/1, Relational Operator2/2
  Add4/1 -> Add5/1, Relational Operator4/2
  [t0] -> Add6/3, Add6/2
  Add3/1 -> Relational Operator3/2, Add4/1
  [t2] -> Add2/2
  [t1] -> Add5/2
  Add5/1 -> Add6/1, Relational Operator5/2
  Add6/1 -> Add7/1, Relational Operator6/2
  Relational Operator11/1 -> Mux/12
  Add1/1 -> Add2/1, Relational Operator1/2
  [t1] -> Add1/2
  Add8/1 -> Add9/1, Relational Operator8/2
  Relational Operator4/1 -> Mux/5
  Add11/1 -> Relational Operator11/2
  Add7/1 -> Add8/1, Relational Operator7/2
  [t0] -> Add3/2
  Relational Operator9/1 -> Mux/10
  Relational Operator2/1 -> Mux/3
  Relational Operator6/1 -> Mux/7
  Relational Operator10/1 -> Mux/11
  Relational Operator7/1 -> Mux/8
  Relational Operator3/1 -> Mux/4
  Mux/1 -> Sum of Elements/1
  d1/1 -> Divide1/1
  d3/1 -> Divide10/1
  d4/1 -> Divide11/1
  d2/1 -> Divide9/1
  Sum of Elements/1 -> Multiport Switch/1
  Multiport Switch/1 -> Out3/1
  d0/1 -> Divide2/1
  Constant5/1 -> Divide2/2
  Divide2/1 -> [t0]
  Constant1/1 -> Divide1/2
  Divide1/1 -> [t1]
  Divide9/1 -> [t2]
  Constant7/1 -> Divide9/2
  Divide10/1 -> [t3]
  Constant10/1 -> Divide10/2
  Divide11/1 -> [t4]
  Constant11/1 -> Divide11/2
  [t3] -> Add7/2
  [t4] -> Add8/2
  [t0] -> Add9/2
  [t4] -> Add10/2
  [t3] -> Add11/2
  v1/1 -> Multiport Switch/7, Multiport Switch/3
  v2/1 -> Multiport Switch/6, Multiport Switch/4
  02/1 -> Multiport Switch/5
  v3/1 -> Multiport Switch/13, Multiport Switch/9
  v4/1 -> Multiport Switch/12, Multiport Switch/10
  03/1 -> Multiport Switch/11
  01/1 -> Multiport Switch/14, Multiport Switch/8, Multiport Switch/2

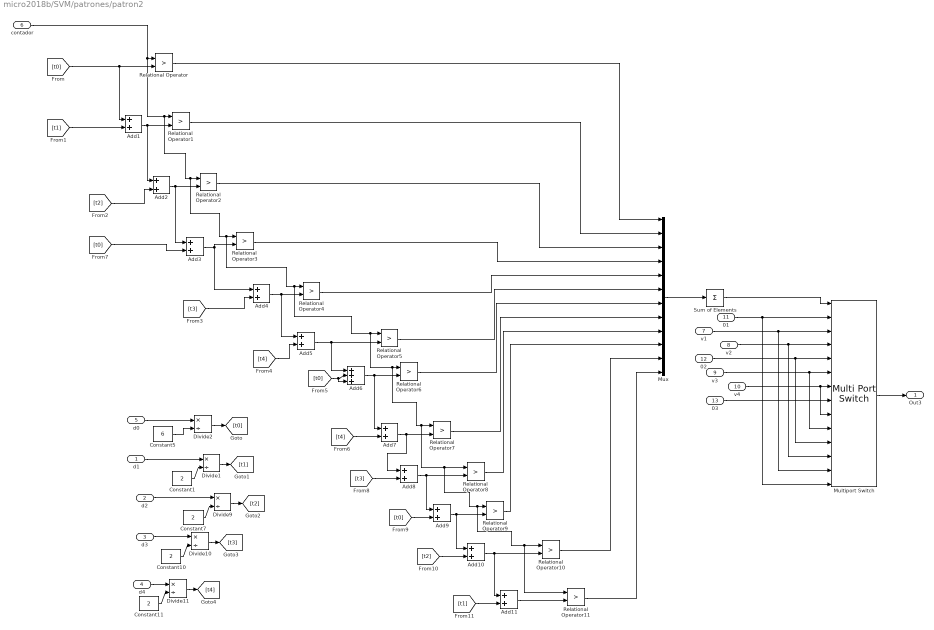
== system micro2018b/SVM/patrones/patron2 ==
  d1 : Inport
  d2 : Inport  Port=2
  d3 : Inport  Port=3
  d4 : Inport  Port=4
  d0 : Inport  Port=5
  contador : Inport  Port=6
  v1 : Inport  Port=7
  v2 : Inport  Port=8
  v3 : Inport  Port=9
  v4 : Inport  Port=10
  01 : Inport  Port=11
  02 : Inport  Port=12
  03 : Inport  Port=13
  Add{1..5,7..11} (10 alike) : Sum
  Add6 : Sum  Inputs=+++
  Constant{1,7,10..11} (4 alike) : Constant  Value=2
  Constant5 : Constant  Value=6
  Divide{1..2,9..11} (5 alike) : Product  Inputs=*/
  Multiport Switch : MultiPortSwitch  DataPortOrder=Zero-based contiguous  Inputs=13  zeroidx=on
  Mux : Mux  Inputs=12
  Relational Operator{,1..11} (12 alike) : RelationalOperator  Operator=>  OutDataTypeStr=boolean  RndMeth=Simplest
  Sum of Elements : Sum  Inputs=+
  Out3 : Outport
  wires:
  contador/1 -> Relational Operator11/1, Relational Operator10/1, Relational Operator9/1, Relational Operator8/1, Relational Operator7/1, Relational Operator6/1, Relational Operator5/1, Relational Operator4/1, Relational Operator3/1, Relational Operator2/1, Relational Operator1/1, Relational Operator/1
  Add10/1 -> Add11/1, Relational Operator10/2
  Add9/1 -> Add10/1, Relational Operator9/2
  [t3] -> Add4/2
  Relational Operator8/1 -> Mux/9
  [t0] -> Add1/1, Relational Operator/2
  Relational Operator/1 -> Mux/1
  Relational Operator1/1 -> Mux/2
  Relational Operator5/1 -> Mux/6
  Add2/1 -> Add3/1, Relational Operator2/2
  Add4/1 -> Add5/1, Relational Operator4/2
  [t0] -> Add6/3, Add6/2
  Add3/1 -> Relational Operator3/2, Add4/1
  [t2] -> Add2/2
  [t4] -> Add5/2
  Add5/1 -> Add6/1, Relational Operator5/2
  Add6/1 -> Add7/1, Relational Operator6/2
  Relational Operator11/1 -> Mux/12
  Add1/1 -> Add2/1, Relational Operator1/2
  [t1] -> Add1/2
  Add8/1 -> Add9/1, Relational Operator8/2
  Relational Operator4/1 -> Mux/5
  Add11/1 -> Relational Operator11/2
  Add7/1 -> Add8/1, Relational Operator7/2
  [t0] -> Add3/2
  Relational Operator9/1 -> Mux/10
  Relational Operator2/1 -> Mux/3
  Relational Operator6/1 -> Mux/7
  Relational Operator10/1 -> Mux/11
  Relational Operator7/1 -> Mux/8
  Relational Operator3/1 -> Mux/4
  Mux/1 -> Sum of Elements/1
  d1/1 -> Divide1/1
  d3/1 -> Divide10/1
  d4/1 -> Divide11/1
  d2/1 -> Divide9/1
  Sum of Elements/1 -> Multiport Switch/1
  Multiport Switch/1 -> Out3/1
  d0/1 -> Divide2/1
  Constant5/1 -> Divide2/2
  Divide2/1 -> [t0]
  Constant1/1 -> Divide1/2
  Divide1/1 -> [t1]
  Divide9/1 -> [t2]
  Constant7/1 -> Divide9/2
  Divide10/1 -> [t3]
  Constant10/1 -> Divide10/2
  Divide11/1 -> [t4]
  Constant11/1 -> Divide11/2
  [t4] -> Add7/2
  [t3] -> Add8/2
  [t0] -> Add9/2
  [t2] -> Add10/2
  [t1] -> Add11/2
  v1/1 -> Multiport Switch/3, Multiport Switch/13
  v2/1 -> Multiport Switch/12, Multiport Switch/4
  02/1 -> Multiport Switch/11, Multiport Switch/5
  01/1 -> Multiport Switch/2, Multiport Switch/14
  v3/1 -> Multiport Switch/10, Multiport Switch/6
  v4/1 -> Multiport Switch/9, Multiport Switch/7
  03/1 -> Multiport Switch/8

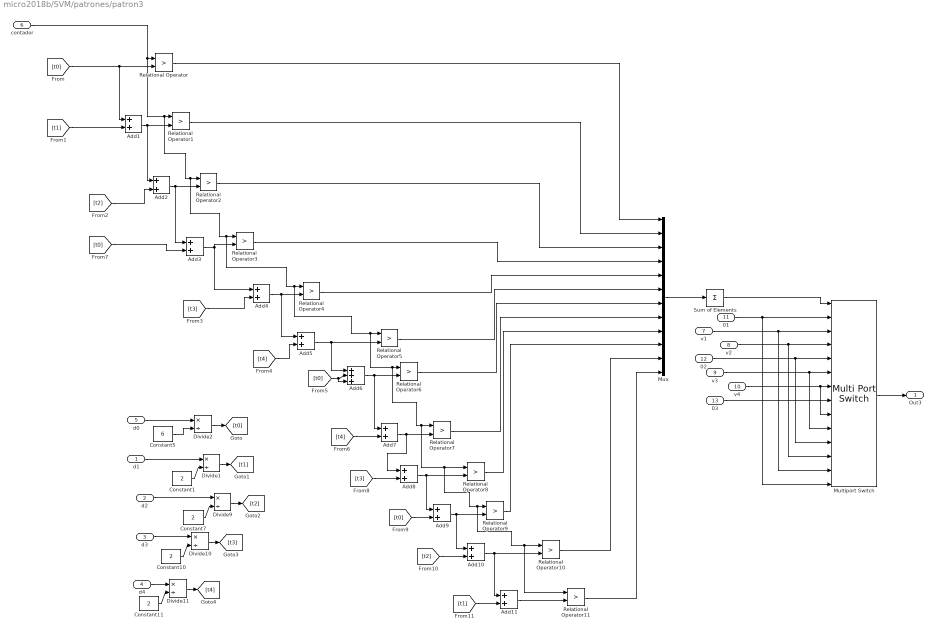
== system micro2018b/SVM/patrones/patron3 ==
  d1 : Inport
  d2 : Inport  Port=2
  d3 : Inport  Port=3
  d4 : Inport  Port=4
  d0 : Inport  Port=5
  contador : Inport  Port=6
  v1 : Inport  Port=7
  v2 : Inport  Port=8
  v3 : Inport  Port=9
  v4 : Inport  Port=10
  01 : Inport  Port=11
  02 : Inport  Port=12
  03 : Inport  Port=13
  Add{1..5,7..11} (10 alike) : Sum
  Add6 : Sum  Inputs=+++
  Constant{1,7,10..11} (4 alike) : Constant  Value=2
  Constant5 : Constant  Value=6
  Divide{1..2,9..11} (5 alike) : Product  Inputs=*/
  Multiport Switch : MultiPortSwitch  DataPortOrder=Zero-based contiguous  Inputs=13  zeroidx=on
  Mux : Mux  Inputs=12
  Relational Operator{,1..11} (12 alike) : RelationalOperator  Operator=>  OutDataTypeStr=boolean  RndMeth=Simplest
  Sum of Elements : Sum  Inputs=+
  Out3 : Outport
  wires:
  contador/1 -> Relational Operator11/1, Relational Operator10/1, Relational Operator9/1, Relational Operator8/1, Relational Operator7/1, Relational Operator6/1, Relational Operator5/1, Relational Operator4/1, Relational Operator3/1, Relational Operator2/1, Relational Operator1/1, Relational Operator/1
  Add10/1 -> Add11/1, Relational Operator10/2
  Add9/1 -> Add10/1, Relational Operator9/2
  [t3] -> Add4/2
  Relational Operator8/1 -> Mux/9
  [t0] -> Add1/1, Relational Operator/2
  Relational Operator/1 -> Mux/1
  Relational Operator1/1 -> Mux/2
  Relational Operator5/1 -> Mux/6
  Add2/1 -> Add3/1, Relational Operator2/2
  Add4/1 -> Add5/1, Relational Operator4/2
  [t0] -> Add6/3, Add6/2
  Add3/1 -> Relational Operator3/2, Add4/1
  [t2] -> Add2/2
  [t4] -> Add5/2
  Add5/1 -> Add6/1, Relational Operator5/2
  Add6/1 -> Add7/1, Relational Operator6/2
  Relational Operator11/1 -> Mux/12
  Add1/1 -> Add2/1, Relational Operator1/2
  [t1] -> Add1/2
  Add8/1 -> Add9/1, Relational Operator8/2
  Relational Operator4/1 -> Mux/5
  Add11/1 -> Relational Operator11/2
  Add7/1 -> Add8/1, Relational Operator7/2
  [t0] -> Add3/2
  Relational Operator9/1 -> Mux/10
  Relational Operator2/1 -> Mux/3
  Relational Operator6/1 -> Mux/7
  Relational Operator10/1 -> Mux/11
  Relational Operator7/1 -> Mux/8
  Relational Operator3/1 -> Mux/4
  Mux/1 -> Sum of Elements/1
  d1/1 -> Divide1/1
  d3/1 -> Divide10/1
  d4/1 -> Divide11/1
  d2/1 -> Divide9/1
  Sum of Elements/1 -> Multiport Switch/1
  Multiport Switch/1 -> Out3/1
  d0/1 -> Divide2/1
  Constant5/1 -> Divide2/2
  Divide2/1 -> [t0]
  Constant1/1 -> Divide1/2
  Divide1/1 -> [t1]
  Divide9/1 -> [t2]
  Constant7/1 -> Divide9/2
  Divide10/1 -> [t3]
  Constant10/1 -> Divide10/2
  Divide11/1 -> [t4]
  Constant11/1 -> Divide11/2
  [t4] -> Add7/2
  [t3] -> Add8/2
  [t0] -> Add9/2
  [t2] -> Add10/2
  [t1] -> Add11/2
  v1/1 -> Multiport Switch/3, Multiport Switch/13
  v2/1 -> Multiport Switch/12, Multiport Switch/4
  02/1 -> Multiport Switch/11, Multiport Switch/5
  01/1 -> Multiport Switch/2, Multiport Switch/14
  v3/1 -> Multiport Switch/10, Multiport Switch/6
  v4/1 -> Multiport Switch/9, Multiport Switch/7
  03/1 -> Multiport Switch/8

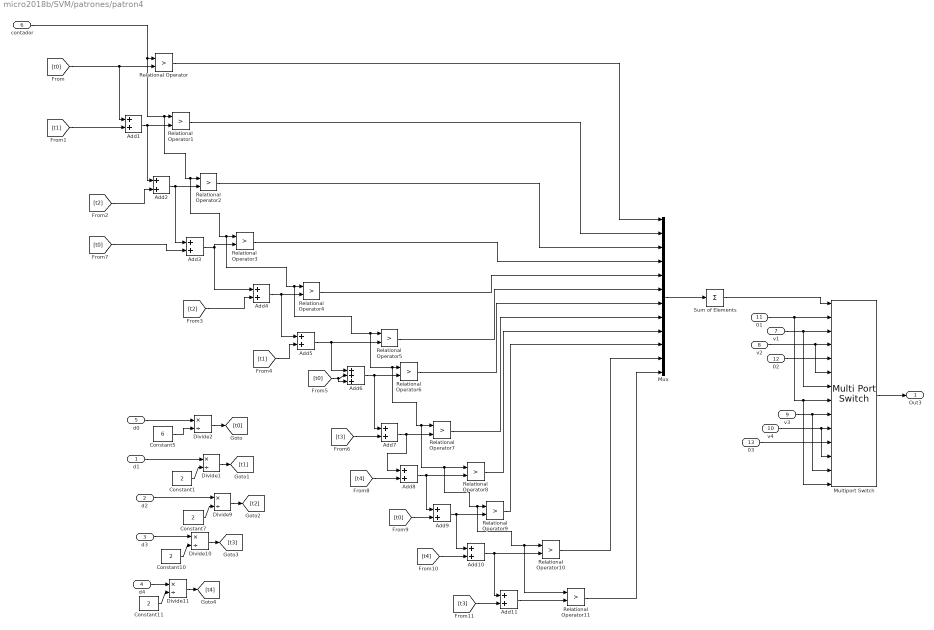
== system micro2018b/SVM/patrones/patron4 ==
  d1 : Inport
  d2 : Inport  Port=2
  d3 : Inport  Port=3
  d4 : Inport  Port=4
  d0 : Inport  Port=5
  contador : Inport  Port=6
  v1 : Inport  Port=7
  v2 : Inport  Port=8
  v3 : Inport  Port=9
  v4 : Inport  Port=10
  01 : Inport  Port=11
  02 : Inport  Port=12
  03 : Inport  Port=13
  Add{1..5,7..11} (10 alike) : Sum
  Add6 : Sum  Inputs=+++
  Constant{1,7,10..11} (4 alike) : Constant  Value=2
  Constant5 : Constant  Value=6
  Divide{1..2,9..11} (5 alike) : Product  Inputs=*/
  Multiport Switch : MultiPortSwitch  DataPortOrder=Zero-based contiguous  Inputs=13  zeroidx=on
  Mux : Mux  Inputs=12
  Relational Operator{,1..11} (12 alike) : RelationalOperator  Operator=>  OutDataTypeStr=boolean  RndMeth=Simplest
  Sum of Elements : Sum  Inputs=+
  Out3 : Outport
  wires:
  contador/1 -> Relational Operator11/1, Relational Operator10/1, Relational Operator9/1, Relational Operator8/1, Relational Operator7/1, Relational Operator6/1, Relational Operator5/1, Relational Operator4/1, Relational Operator3/1, Relational Operator2/1, Relational Operator1/1, Relational Operator/1
  Add10/1 -> Add11/1, Relational Operator10/2
  Add9/1 -> Add10/1, Relational Operator9/2
  [t2] -> Add4/2
  Relational Operator8/1 -> Mux/9
  [t0] -> Add1/1, Relational Operator/2
  Relational Operator/1 -> Mux/1
  Relational Operator1/1 -> Mux/2
  Relational Operator5/1 -> Mux/6
  Add2/1 -> Add3/1, Relational Operator2/2
  Add4/1 -> Add5/1, Relational Operator4/2
  [t0] -> Add6/3, Add6/2
  Add3/1 -> Relational Operator3/2, Add4/1
  [t2] -> Add2/2
  [t1] -> Add5/2
  Add5/1 -> Add6/1, Relational Operator5/2
  Add6/1 -> Add7/1, Relational Operator6/2
  Relational Operator11/1 -> Mux/12
  Add1/1 -> Add2/1, Relational Operator1/2
  [t1] -> Add1/2
  Add8/1 -> Add9/1, Relational Operator8/2
  Relational Operator4/1 -> Mux/5
  Add11/1 -> Relational Operator11/2
  Add7/1 -> Add8/1, Relational Operator7/2
  [t0] -> Add3/2
  Relational Operator9/1 -> Mux/10
  Relational Operator2/1 -> Mux/3
  Relational Operator6/1 -> Mux/7
  Relational Operator10/1 -> Mux/11
  Relational Operator7/1 -> Mux/8
  Relational Operator3/1 -> Mux/4
  Mux/1 -> Sum of Elements/1
  d1/1 -> Divide1/1
  d3/1 -> Divide10/1
  d4/1 -> Divide11/1
  d2/1 -> Divide9/1
  Sum of Elements/1 -> Multiport Switch/1
  Multiport Switch/1 -> Out3/1
  d0/1 -> Divide2/1
  Constant5/1 -> Divide2/2
  Divide2/1 -> [t0]
  Constant1/1 -> Divide1/2
  Divide1/1 -> [t1]
  Divide9/1 -> [t2]
  Constant7/1 -> Divide9/2
  Divide10/1 -> [t3]
  Constant10/1 -> Divide10/2
  Divide11/1 -> [t4]
  Constant11/1 -> Divide11/2
  [t3] -> Add7/2
  [t4] -> Add8/2
  [t0] -> Add9/2
  [t4] -> Add10/2
  [t3] -> Add11/2
  v1/1 -> Multiport Switch/7, Multiport Switch/3
  v2/1 -> Multiport Switch/6, Multiport Switch/4
  02/1 -> Multiport Switch/5
  v3/1 -> Multiport Switch/13, Multiport Switch/9
  v4/1 -> Multiport Switch/12, Multiport Switch/10
  03/1 -> Multiport Switch/11
  01/1 -> Multiport Switch/14, Multiport Switch/8, Multiport Switch/2

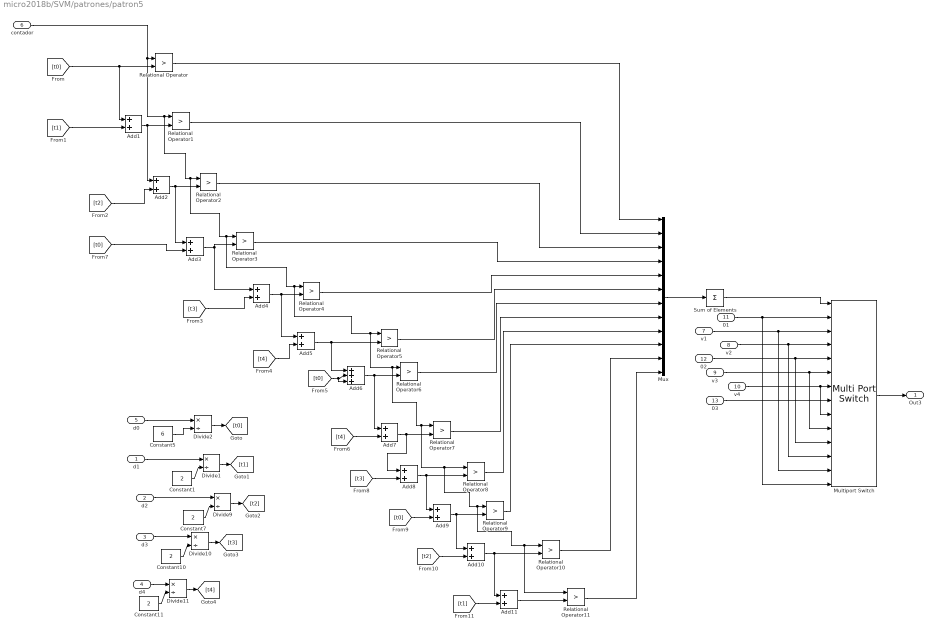
== system micro2018b/SVM/patrones/patron5 ==
  d1 : Inport
  d2 : Inport  Port=2
  d3 : Inport  Port=3
  d4 : Inport  Port=4
  d0 : Inport  Port=5
  contador : Inport  Port=6
  v1 : Inport  Port=7
  v2 : Inport  Port=8
  v3 : Inport  Port=9
  v4 : Inport  Port=10
  01 : Inport  Port=11
  02 : Inport  Port=12
  03 : Inport  Port=13
  Add{1..5,7..11} (10 alike) : Sum
  Add6 : Sum  Inputs=+++
  Constant{1,7,10..11} (4 alike) : Constant  Value=2
  Constant5 : Constant  Value=6
  Divide{1..2,9..11} (5 alike) : Product  Inputs=*/
  Multiport Switch : MultiPortSwitch  DataPortOrder=Zero-based contiguous  Inputs=13  zeroidx=on
  Mux : Mux  Inputs=12
  Relational Operator{,1..11} (12 alike) : RelationalOperator  Operator=>  OutDataTypeStr=boolean  RndMeth=Simplest
  Sum of Elements : Sum  Inputs=+
  Out3 : Outport
  wires:
  contador/1 -> Relational Operator11/1, Relational Operator10/1, Relational Operator9/1, Relational Operator8/1, Relational Operator7/1, Relational Operator6/1, Relational Operator5/1, Relational Operator4/1, Relational Operator3/1, Relational Operator2/1, Relational Operator1/1, Relational Operator/1
  Add10/1 -> Add11/1, Relational Operator10/2
  Add9/1 -> Add10/1, Relational Operator9/2
  [t3] -> Add4/2
  Relational Operator8/1 -> Mux/9
  [t0] -> Add1/1, Relational Operator/2
  Relational Operator/1 -> Mux/1
  Relational Operator1/1 -> Mux/2
  Relational Operator5/1 -> Mux/6
  Add2/1 -> Add3/1, Relational Operator2/2
  Add4/1 -> Add5/1, Relational Operator4/2
  [t0] -> Add6/3, Add6/2
  Add3/1 -> Relational Operator3/2, Add4/1
  [t2] -> Add2/2
  [t4] -> Add5/2
  Add5/1 -> Add6/1, Relational Operator5/2
  Add6/1 -> Add7/1, Relational Operator6/2
  Relational Operator11/1 -> Mux/12
  Add1/1 -> Add2/1, Relational Operator1/2
  [t1] -> Add1/2
  Add8/1 -> Add9/1, Relational Operator8/2
  Relational Operator4/1 -> Mux/5
  Add11/1 -> Relational Operator11/2
  Add7/1 -> Add8/1, Relational Operator7/2
  [t0] -> Add3/2
  Relational Operator9/1 -> Mux/10
  Relational Operator2/1 -> Mux/3
  Relational Operator6/1 -> Mux/7
  Relational Operator10/1 -> Mux/11
  Relational Operator7/1 -> Mux/8
  Relational Operator3/1 -> Mux/4
  Mux/1 -> Sum of Elements/1
  d1/1 -> Divide1/1
  d3/1 -> Divide10/1
  d4/1 -> Divide11/1
  d2/1 -> Divide9/1
  Sum of Elements/1 -> Multiport Switch/1
  Multiport Switch/1 -> Out3/1
  d0/1 -> Divide2/1
  Constant5/1 -> Divide2/2
  Divide2/1 -> [t0]
  Constant1/1 -> Divide1/2
  Divide1/1 -> [t1]
  Divide9/1 -> [t2]
  Constant7/1 -> Divide9/2
  Divide10/1 -> [t3]
  Constant10/1 -> Divide10/2
  Divide11/1 -> [t4]
  Constant11/1 -> Divide11/2
  [t4] -> Add7/2
  [t3] -> Add8/2
  [t0] -> Add9/2
  [t2] -> Add10/2
  [t1] -> Add11/2
  v1/1 -> Multiport Switch/3, Multiport Switch/13
  v2/1 -> Multiport Switch/12, Multiport Switch/4
  02/1 -> Multiport Switch/11, Multiport Switch/5
  01/1 -> Multiport Switch/2, Multiport Switch/14
  v3/1 -> Multiport Switch/10, Multiport Switch/6
  v4/1 -> Multiport Switch/9, Multiport Switch/7
  03/1 -> Multiport Switch/8

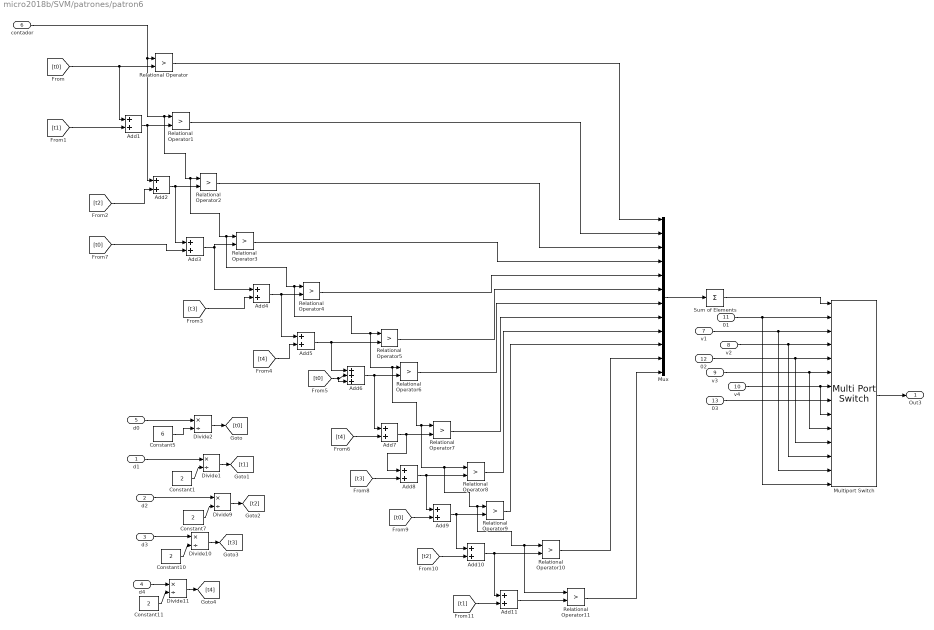
== system micro2018b/SVM/patrones/patron6 ==
  d1 : Inport
  d2 : Inport  Port=2
  d3 : Inport  Port=3
  d4 : Inport  Port=4
  d0 : Inport  Port=5
  contador : Inport  Port=6
  v1 : Inport  Port=7
  v2 : Inport  Port=8
  v3 : Inport  Port=9
  v4 : Inport  Port=10
  01 : Inport  Port=11
  02 : Inport  Port=12
  03 : Inport  Port=13
  Add{1..5,7..11} (10 alike) : Sum
  Add6 : Sum  Inputs=+++
  Constant{1,7,10..11} (4 alike) : Constant  Value=2
  Constant5 : Constant  Value=6
  Divide{1..2,9..11} (5 alike) : Product  Inputs=*/
  Multiport Switch : MultiPortSwitch  DataPortOrder=Zero-based contiguous  Inputs=13  zeroidx=on
  Mux : Mux  Inputs=12
  Relational Operator{,1..11} (12 alike) : RelationalOperator  Operator=>  OutDataTypeStr=boolean  RndMeth=Simplest
  Sum of Elements : Sum  Inputs=+
  Out3 : Outport
  wires:
  contador/1 -> Relational Operator11/1, Relational Operator10/1, Relational Operator9/1, Relational Operator8/1, Relational Operator7/1, Relational Operator6/1, Relational Operator5/1, Relational Operator4/1, Relational Operator3/1, Relational Operator2/1, Relational Operator1/1, Relational Operator/1
  Add10/1 -> Add11/1, Relational Operator10/2
  Add9/1 -> Add10/1, Relational Operator9/2
  [t3] -> Add4/2
  Relational Operator8/1 -> Mux/9
  [t0] -> Add1/1, Relational Operator/2
  Relational Operator/1 -> Mux/1
  Relational Operator1/1 -> Mux/2
  Relational Operator5/1 -> Mux/6
  Add2/1 -> Add3/1, Relational Operator2/2
  Add4/1 -> Add5/1, Relational Operator4/2
  [t0] -> Add6/3, Add6/2
  Add3/1 -> Relational Operator3/2, Add4/1
  [t2] -> Add2/2
  [t4] -> Add5/2
  Add5/1 -> Add6/1, Relational Operator5/2
  Add6/1 -> Add7/1, Relational Operator6/2
  Relational Operator11/1 -> Mux/12
  Add1/1 -> Add2/1, Relational Operator1/2
  [t1] -> Add1/2
  Add8/1 -> Add9/1, Relational Operator8/2
  Relational Operator4/1 -> Mux/5
  Add11/1 -> Relational Operator11/2
  Add7/1 -> Add8/1, Relational Operator7/2
  [t0] -> Add3/2
  Relational Operator9/1 -> Mux/10
  Relational Operator2/1 -> Mux/3
  Relational Operator6/1 -> Mux/7
  Relational Operator10/1 -> Mux/11
  Relational Operator7/1 -> Mux/8
  Relational Operator3/1 -> Mux/4
  Mux/1 -> Sum of Elements/1
  d1/1 -> Divide1/1
  d3/1 -> Divide10/1
  d4/1 -> Divide11/1
  d2/1 -> Divide9/1
  Sum of Elements/1 -> Multiport Switch/1
  Multiport Switch/1 -> Out3/1
  d0/1 -> Divide2/1
  Constant5/1 -> Divide2/2
  Divide2/1 -> [t0]
  Constant1/1 -> Divide1/2
  Divide1/1 -> [t1]
  Divide9/1 -> [t2]
  Constant7/1 -> Divide9/2
  Divide10/1 -> [t3]
  Constant10/1 -> Divide10/2
  Divide11/1 -> [t4]
  Constant11/1 -> Divide11/2
  [t4] -> Add7/2
  [t3] -> Add8/2
  [t0] -> Add9/2
  [t2] -> Add10/2
  [t1] -> Add11/2
  v1/1 -> Multiport Switch/3, Multiport Switch/13
  v2/1 -> Multiport Switch/12, Multiport Switch/4
  02/1 -> Multiport Switch/11, Multiport Switch/5
  01/1 -> Multiport Switch/2, Multiport Switch/14
  v3/1 -> Multiport Switch/10, Multiport Switch/6
  v4/1 -> Multiport Switch/9, Multiport Switch/7
  03/1 -> Multiport Switch/8

== system micro2018b/SVM/patrones/ticks_calculator ==
  d1 : Inport
  d2 : Inport  Port=2
  d3 : Inport  Port=3
  d4 : Inport  Port=4
  ticks_per_period : Inport  Port=5
  Add : Sum  Inputs=----+
  Product{,1..3} (4 alike) : Product
  Out1 : Outport
  Out2 : Outport  Port=2
  Out3 : Outport  Port=3
  Out4 : Outport  Port=4
  d0 : Outport  Port=5
  wires:
  Product2/1 -> Add/3, Out3/1
  ticks_per_period/1 -> Add/5, Product/2, Product1/2, Product2/2, Product3/2
  Product/1 -> Out1/1, Add/1
  d1/1 -> Product/1
  Product3/1 -> Add/4, Out4/1
  d3/1 -> Product2/1
  Product1/1 -> Add/2, Out2/1
  d2/1 -> Product1/1
  d4/1 -> Product3/1
  Add/1 -> d0/1
